simulink model "transmitComplexEnvelopeFromWorkspace_USRP"  (R2017a)
settings: Solver=ode45  StartTime=0.0  StopTime=inf  RelTol=1e-3  EnableMultiTasking=on
libraries: commsdrhw_v2 x1, dspsrcs4 x1
settings Model: Creator=prust  LastModifiedBy=prust
settings DataIOCC: SaveFormat=Array  SaveOutput=off  SignalLogging=off  DSMLogging=off  VisualizeSimOutput=off  SaveTime=off
settings OptimizationCC: LifeSpan=inf
settings DebuggingCC: SFUnexpectedBacktrackingDiag=warning  SFNoUnconditionalDefaultTransitionDiag=warning  SFExecutionAtInitializationDiag=none
settings HardwareCC: ProdBitPerPointer=32  ProdBitPerSizeT=32  ProdBitPerPtrDiffT=32  ProdLargestAtomicFloat=None  ProdIntDivRoundTo=Undefined  ProdEndianess=Unspecified  ProdWordSize=32  ProdHWDeviceType=32-bit Generic
settings ModelReferenceCC: PropagateSignalLabelsOutOfModel=off
settings GRTTargetCC: TargetLangStandard=C89/C90 (ANSI)  GeneratePreprocessorConditionals=Disable all
settings ConfigComp: CovMetricSettings=dw  CovHtmlReporting=on  CovSaveCumulativeToWorkspaceVar=on  CovSaveSingleToWorkspaceVar=on  CovExternalEMLEnable=off

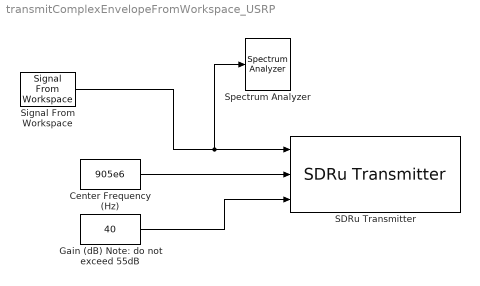
== system transmitComplexEnvelopeFromWorkspace_USRP ==
  Center Frequency (Hz) : Constant  Value=905e6  SampleTime=-1
  Gain (dB) Note: do not exceed 55dB : Constant  Value=40  SampleTime=-1
  SDRu Transmitter : commsdrhw_v2/SDRu Transmitter  SourceLibraryInfo="This block requires <a href=\"http://www.mathworks.com/hardware-support/usrp.html\">Communications System Toolbox Support Package for USRP Radio</a>"  rxtx=tx  platform=B200  USRP2_IP='192.168.10.2'  USRP_IP_X300='192.168.10.2'  USRP_IP_X310='192.168.10.2'  USRP_serialNumB200='30703A1'  USRP_serialNumB210='307346D'  ChannelMapping=1  centerFrequency=900e6  centerFrequencySrc=Input port  loOffset=0  loOffsetSrc=Dialog  PPSSource=Internal  clockSource=Internal  masterClkRateB200=24e6  masterClkRateB210=24e6  masterClkRateX300=200e6  masterClkRateX310=200e6  masterClkRateParam=24000000  gain=50  gainSrc=Input port  decimInterp=100  decimInterpSrc=Dialog  TransportDataType=int16  USRP2_IP_NUM=[51 48 55 48 51 65 49]  frameLength=362  outputDatatype=Same as transport data type  overrunUnderrunPort=off  sampleTime=1  dboardInfo=|  HOST_DATA_PORT=30000  HOST_CONTROL_PORT=30001  USRP2_DATA_PORT=32769  USRP2_CONTROL_PORT=32768  bufferMode=Continuous streaming  EnableBurstMode=off  NumFramesInBurst=100  USRP_ID='30703A1'
      | dbid: 0
      |           dbName: 'no db found'
      |          freqMin: 0
      |          freqMax: 0
      |          gainMin: 0
      |          gainMax: 0
      |     gainStepSize: 0
      settings: SourceProductName=Communications System Toolbox Support Package for USRP(R) Radio  SourceProductBaseCode=USRP
  Signal From Workspace : dspsrcs4/Signal From Workspace  X=z  Ts=1/240e3  nsamps=1000  OutputAfterFinalValue=Cyclic repetition  ignoreOrWarnInputAndFrameLengths=off  OutputFrames=on
  Spectrum Analyzer : SpectrumAnalyzer
  wires:
  Center Frequency (Hz)/1 -> SDRu Transmitter/2
  Signal From Workspace/1 -> Spectrum Analyzer/1, SDRu Transmitter/1
  Gain (dB) Note: do not exceed 55dB/1 -> SDRu Transmitter/3
